simulink model "as_labor04_hbridge"  (R2020b)
settings: Solver=ode15s  StartTime=0.0  StopTime=7  RelTol=1e-3
values from neighbouring files (symbols this model uses):
  cr = km*1/m    [as_labor02_2.m]    (also in as_labor03_const_u_motor_dc.m = 3.24086977369e-07; as_labor04_hbridge.m = 3.24086977369e-07)
  i_minus = -0.01    [as_labor04_hbridge.m]
  i_plus = 0.01    [as_labor04_hbridge.m]
  J = 0.000005    (= 5e-06)    [as_labor03_const_u_motor_dc.m]    (also in as_labor04_hbridge.m)
  ke = 0.023520507251362    (= 0.0235205072514)    [as_labor03_const_u_motor_dc.m]    (also in as_labor04_hbridge.m)
  km = 0.022031575949394    (= 0.0220315759494)    [as_labor02_2.m]    (also in as_labor03_const_u_motor_dc.m; as_labor04_hbridge.m)
  L = 1.754462619198655e-04    (= 0.00017544626192)    [RLC_M.m]    (also in as_labor03_const_u_motor_dc.m; as_labor04_hbridge.m)
  R = 3.263586106324851    (= 3.26358610632)    [RLC_M.m]    (also in as_labor01_2.m = 1/f2(1,1); as_labor03_const_u_motor_dc.m; as_labor04_hbridge.m)
  Rs = 1    [as_labor03_const_u_motor_dc.m]    (also in as_labor04_hbridge.m)
  U_D = 0.7    [as_labor04_hbridge.m]
  U_H = 15    [as_labor04_hbridge.m]
settings Model: SimulationMode=rapid-accelerator  Creator=jan  LastModifiedBy=jan
settings HardwareCC: ProdBitPerLong=64  ProdHWDeviceType=Intel->x86-64 (Linux 64)

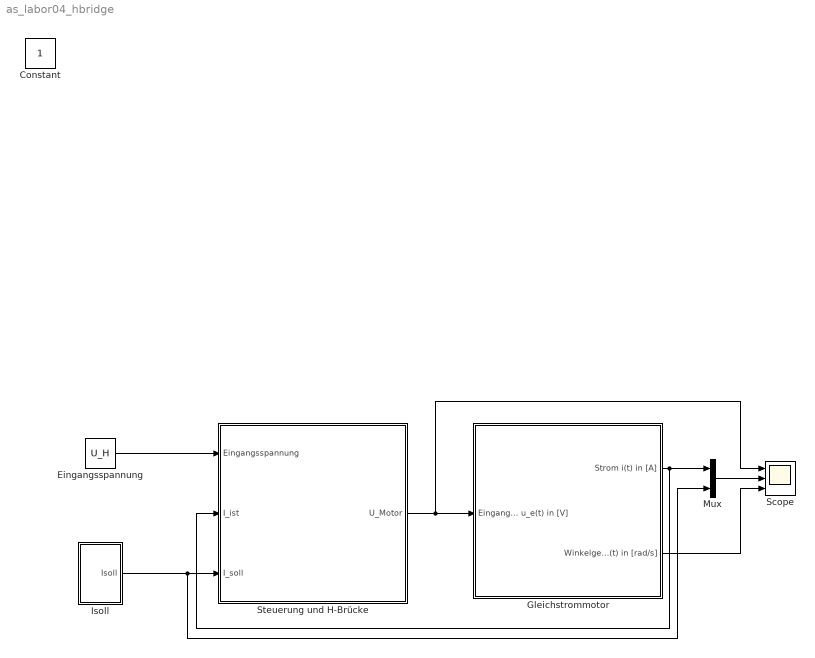
== system as_labor04_hbridge ==
  Eingangsspannung : Constant  Value=U_H
  Gleichstrommotor : Subsystem
  Isoll : Subsystem
  Mux : Mux  Inputs=2
  Scope : Scope  NumInputPorts=3
  Steuerung und H-Brücke : Subsystem
  Constant : Constant  IOType=siggen
  wires:
  Gleichstrommotor/1(Strom i(t) in [A]) -> Mux/1, Steuerung und H-Brücke/2(I_ist)
  Gleichstrommotor/2(Winkelgeschwindigkeit w(t) in [rad/s]) -> Scope/3
  Steuerung und H-Brücke/1(U_Motor) -> Scope/1, Gleichstrommotor/1(Eingangspannung u_e(t) in [V])
  Isoll/1(Isoll) -> Mux/2, Steuerung und H-Brücke/3(I_soll)
  Eingangsspannung/1 -> Steuerung und H-Brücke/1(Eingangsspannung)
  Mux/1 -> Scope/2

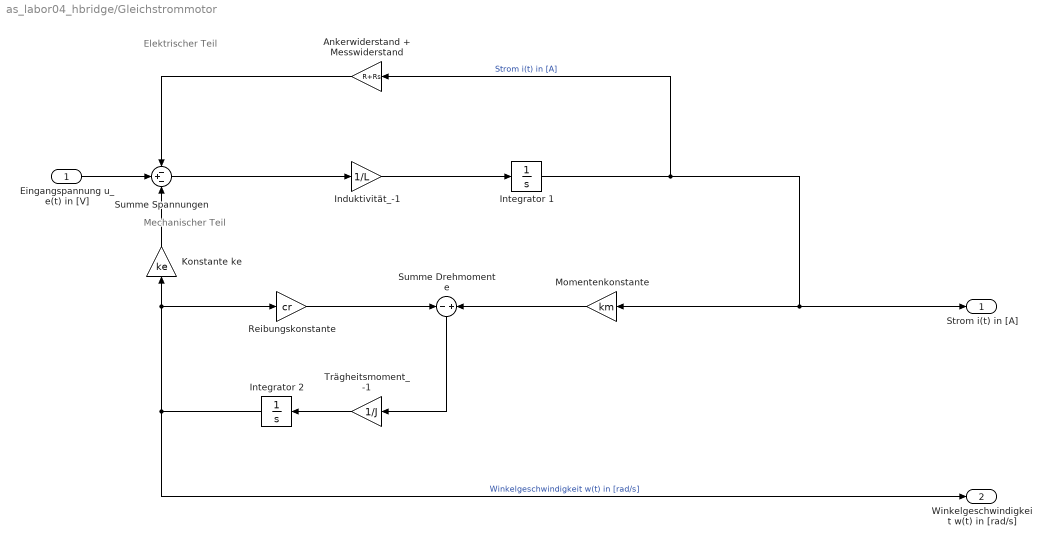
== system as_labor04_hbridge/Gleichstrommotor ==
  note: Elektrischer Teil
  note: Mechanischer Teil
  Eingangspannung u_e(t) in [V] : Inport
  Ankerwiderstand + Messwiderstand : Gain  Gain=R+Rs
  Induktivität_-1 : Gain  Gain=1/L
  Integrator 1 : Integrator
  Integrator 2 : Integrator
  Konstante ke : Gain  Gain=ke
  Momentenkonstante : Gain  Gain=km
  Reibungskonstante : Gain  Gain=cr
  Summe Drehmomente : Sum  Inputs=-|+
  Summe Spannungen : Sum  Inputs=-+-
  Trägheitsmoment_-1 : Gain  Gain=1/J
  Strom i(t) in [A] : Outport
  Winkelgeschwindigkeit w(t) in [rad/s] : Outport  Port=2
  wires:
  Ankerwiderstand + Messwiderstand/1 -> Summe Spannungen/1
  Reibungskonstante/1 -> Summe Drehmomente/1
  Integrator 2/1 -> Winkelgeschwindigkeit w(t) in [rad/s]/1, Reibungskonstante/1, Konstante ke/1  "Winkelgeschwindigkeit w(t) in [rad/s]"
  Summe Drehmomente/1 -> Trägheitsmoment_-1/1
  Eingangspannung u_e(t) in [V]/1 -> Summe Spannungen/2
  Integrator 1/1 -> Momentenkonstante/1, Strom i(t) in [A]/1, Ankerwiderstand + Messwiderstand/1  "Strom i(t) in [A]"
  Trägheitsmoment_-1/1 -> Integrator 2/1
  Konstante ke/1 -> Summe Spannungen/3
  Momentenkonstante/1 -> Summe Drehmomente/2
  Induktivität_-1/1 -> Integrator 1/1
  Summe Spannungen/1 -> Induktivität_-1/1

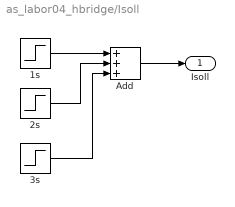
== system as_labor04_hbridge/Isoll ==
  1s : Step  Time=0  After=0.5  SampleTime=0.01
  2s : Step  Time=2  After=-0.8  SampleTime=0.01
  3s : Step  Time=4  After=0.9  SampleTime=0.01
  Add : Sum  Inputs=+++
  Isoll : Outport
  wires:
  3s/1 -> Add/3
  2s/1 -> Add/2
  1s/1 -> Add/1
  Add/1 -> Isoll/1

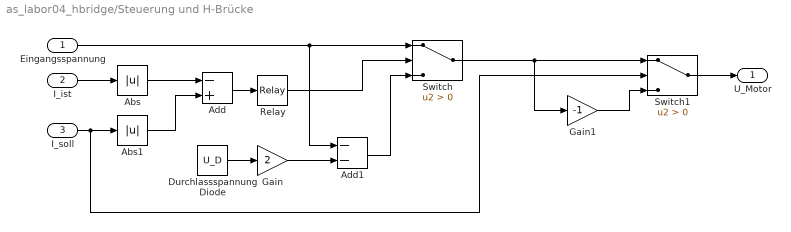
== system as_labor04_hbridge/Steuerung und H-Brücke ==
  Eingangsspannung : Inport
  I_ist : Inport  Port=2
  I_soll : Inport  Port=3
  Abs : Abs
  Abs1 : Abs
  Add : Sum  Inputs=-+
  Add1 : Sum  Inputs=--
  Durchlassspannung Diode : Constant  Value=U_D
  Gain : Gain  Gain=2
  Gain1 : Gain  Gain=-1
  Relay : Relay  OnSwitchValue=i_plus  OffSwitchValue=i_minus
  Switch : Switch  Criteria=u2 > Threshold
  Switch1 : Switch  Criteria=u2 > Threshold
  U_Motor : Outport
  wires:
  Abs1/1 -> Add/2
  Durchlassspannung Diode/1 -> Gain/1
  Relay/1 -> Switch/2
  Add/1 -> Relay/1
  Add1/1 -> Switch/3
  Abs/1 -> Add/1
  I_soll/1 -> Switch1/2, Abs1/1
  I_ist/1 -> Abs/1
  Eingangsspannung/1 -> Add1/1, Switch/1
  Gain/1 -> Add1/2
  Switch/1 -> Gain1/1, Switch1/1
  Gain1/1 -> Switch1/3
  Switch1/1 -> U_Motor/1
